simulink model "pid"  (R2022a)
settings: Solver=VariableStepAuto  StartTime=0  StopTime=15  RelTol=1e-3
libraries: slpidlib x3
settings Model: Creator=yfx13  LastModifiedBy=yfx13

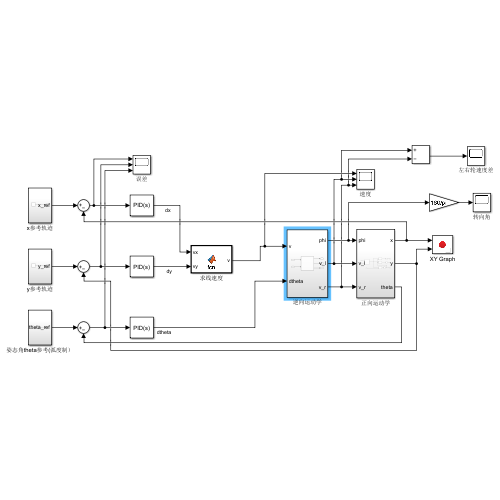
[thumbnail: Simulink's stored preview of the top-level diagram]
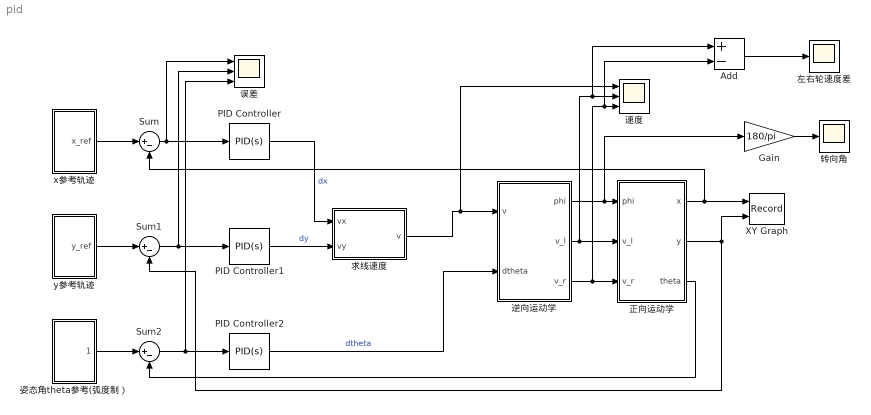
== system pid ==
  Add : Sum  Inputs=+-
  Gain : Gain  Gain=180/pi
  PID Controller : slpidlib/PID Controller  Controller=PID  Form=Parallel  TimeDomain=Continuous-time  UseExternalTs=off  SampleTime=-1  IntegratorMethod=Forward Euler  FilterMethod=Forward Euler  ControllerParametersSource=internal  P=11.7  I=0.72  UseKiTs=off  D=0.86  N=100  UseFilter=on  TunerSelectOption=Transfer Function Based (PID Tuner App)  InitialConditionSource=internal  InitialConditionForIntegrator=0  InitialConditionForFilter=0  DifferentiatorICPrevScaledInput=0  ExternalReset=none  TrackingMode=off  Kt=1  LimitOutput=off  SatLimitsSource=internal  UpperSaturationLimit=inf  LowerSaturationLimit=-inf  LinearizeAsGain=on  AntiWindupMode=none  Kb=1  POutMin=[]  POutMax=[]  IOutMin=[]  IOutMax=[]  DOutMin=[]  DOutMax=[]  NOutMin=[]  NOutMax=[]  SumOutMin=[]  SumOutMax=[]  SaturationOutMin=[]  SaturationOutMax=[]  PParamMin=[]  PParamMax=[]  IParamMin=[]  IParamMax=[]  DParamMin=[]  DParamMax=[]  NParamMin=[]  NParamMax=[]  KbParamMin=[]  KbParamMax=[]  KtParamMin=[]  KtParamMax=[]  KbOutMin=[]  KbOutMax=[]  KtOutMin=[]  KtOutMax=[]  IntegratorOutMin=[]  IntegratorOutMax=[]  FilterOutMin=[]  FilterOutMax=[]  SumI1OutMin=[]  SumI1OutMax=[]  SumI2OutMin=[]  SumI2OutMax=[]  SumI3OutMin=[]  SumI3OutMax=[]  SumI4OutMin=[]  SumI4OutMax=[]  SumDOutMin=[]  SumDOutMax=[]  DifferentiatorOutMin=[]  DifferentiatorOutMax=[]  FilterDiffOutCoefMin=[]  FilterDiffOutCoefMax=[]  ReciprocalOutMin=[]  ReciprocalOutMax=[]  SumDenOutMin=[]  SumDenOutMax=[]  SumNumOutMin=[]  SumNumOutMax=[]  DivideOutMin=[]  DivideOutMax=[]  UdiffTsProdOutMin=[]  UdiffTsProdOutMax=[]  NTsProdOutMin=[]  NTsProdOutMax=[]  UintegralTsProdOutMin=[]  UintegralTsProdOutMax=[]  UngainTsProdOutMin=[]  UngainTsProdOutMax=[]  IntegratorContinuousStateAttributes=''  IntegratorStateMustResolveToSignalObject=off  IntegratorRTWStateStorageClass=Auto  FilterContinuousStateAttributes=''  FilterStateMustResolveToSignalObject=off  FilterRTWStateStorageClass=Auto  ParallelPVariant=InternalParameters  IdealPVariant=Disabled  IVariant=InternalParameters  DVariant=InternalParameters  IntegratorVariant=Continuous  SatVariant=Disabled  AWVariant=Passthrough  PCopyVariant=Disabled  TRVariant=Disabled  FdbkBlocksVariant=Forward  IdealPFdbkVariant=Disabled  SatFdbkVariant=Disabled  DerivativeFilterVariant=ContFilter  NVariant=InternalParameters  NCopyVariant=Disabled  FilterICVariant=InternalICsFilter  IntegratorICVariant=InternalICs  ExternalResetVariant=Disabled  TRSumVariant=Passthrough  SumFdbkVariant=Disabled  SumVariant=Sum_PID  TsampFilterVariant=InternalTs  TsampNgainVariant=Passthrough  TsampIntegralVariant=Passthrough  ExternalSaturationOutDataTypeStr=Inherit: Same as second input  aMode=0
  PID Controller1 : slpidlib/PID Controller  Controller=PID  Form=Parallel  TimeDomain=Continuous-time  UseExternalTs=off  SampleTime=-1  IntegratorMethod=Forward Euler  FilterMethod=Forward Euler  ControllerParametersSource=internal  P=11.6  I=0.63  UseKiTs=off  D=0.78  N=100  UseFilter=on  TunerSelectOption=Transfer Function Based (PID Tuner App)  InitialConditionSource=internal  InitialConditionForIntegrator=0  InitialConditionForFilter=0  DifferentiatorICPrevScaledInput=0  ExternalReset=none  TrackingMode=off  Kt=1  LimitOutput=off  SatLimitsSource=internal  UpperSaturationLimit=inf  LowerSaturationLimit=-inf  LinearizeAsGain=on  AntiWindupMode=none  Kb=1  POutMin=[]  POutMax=[]  IOutMin=[]  IOutMax=[]  DOutMin=[]  DOutMax=[]  NOutMin=[]  NOutMax=[]  SumOutMin=[]  SumOutMax=[]  SaturationOutMin=[]  SaturationOutMax=[]  PParamMin=[]  PParamMax=[]  IParamMin=[]  IParamMax=[]  DParamMin=[]  DParamMax=[]  NParamMin=[]  NParamMax=[]  KbParamMin=[]  KbParamMax=[]  KtParamMin=[]  KtParamMax=[]  KbOutMin=[]  KbOutMax=[]  KtOutMin=[]  KtOutMax=[]  IntegratorOutMin=[]  IntegratorOutMax=[]  FilterOutMin=[]  FilterOutMax=[]  SumI1OutMin=[]  SumI1OutMax=[]  SumI2OutMin=[]  SumI2OutMax=[]  SumI3OutMin=[]  SumI3OutMax=[]  SumI4OutMin=[]  SumI4OutMax=[]  SumDOutMin=[]  SumDOutMax=[]  DifferentiatorOutMin=[]  DifferentiatorOutMax=[]  FilterDiffOutCoefMin=[]  FilterDiffOutCoefMax=[]  ReciprocalOutMin=[]  ReciprocalOutMax=[]  SumDenOutMin=[]  SumDenOutMax=[]  SumNumOutMin=[]  SumNumOutMax=[]  DivideOutMin=[]  DivideOutMax=[]  UdiffTsProdOutMin=[]  UdiffTsProdOutMax=[]  NTsProdOutMin=[]  NTsProdOutMax=[]  UintegralTsProdOutMin=[]  UintegralTsProdOutMax=[]  UngainTsProdOutMin=[]  UngainTsProdOutMax=[]  IntegratorContinuousStateAttributes=''  IntegratorStateMustResolveToSignalObject=off  IntegratorRTWStateStorageClass=Auto  FilterContinuousStateAttributes=''  FilterStateMustResolveToSignalObject=off  FilterRTWStateStorageClass=Auto  ParallelPVariant=InternalParameters  IdealPVariant=Disabled  IVariant=InternalParameters  DVariant=InternalParameters  IntegratorVariant=Continuous  SatVariant=Disabled  AWVariant=Passthrough  PCopyVariant=Disabled  TRVariant=Disabled  FdbkBlocksVariant=Forward  IdealPFdbkVariant=Disabled  SatFdbkVariant=Disabled  DerivativeFilterVariant=ContFilter  NVariant=InternalParameters  NCopyVariant=Disabled  FilterICVariant=InternalICsFilter  IntegratorICVariant=InternalICs  ExternalResetVariant=Disabled  TRSumVariant=Passthrough  SumFdbkVariant=Disabled  SumVariant=Sum_PID  TsampFilterVariant=InternalTs  TsampNgainVariant=Passthrough  TsampIntegralVariant=Passthrough  ExternalSaturationOutDataTypeStr=Inherit: Same as second input  aMode=0
  PID Controller2 : slpidlib/PID Controller  Controller=PID  Form=Parallel  TimeDomain=Continuous-time  UseExternalTs=off  SampleTime=-1  IntegratorMethod=Forward Euler  FilterMethod=Forward Euler  ControllerParametersSource=internal  P=10.3  I=2.86  UseKiTs=off  D=0.028  N=100  UseFilter=on  TunerSelectOption=Transfer Function Based (PID Tuner App)  InitialConditionSource=internal  InitialConditionForIntegrator=0.001  InitialConditionForFilter=0  DifferentiatorICPrevScaledInput=0  ExternalReset=none  TrackingMode=off  Kt=1  LimitOutput=off  SatLimitsSource=internal  UpperSaturationLimit=inf  LowerSaturationLimit=-inf  LinearizeAsGain=on  AntiWindupMode=none  Kb=1  POutMin=[]  POutMax=[]  IOutMin=[]  IOutMax=[]  DOutMin=[]  DOutMax=[]  NOutMin=[]  NOutMax=[]  SumOutMin=[]  SumOutMax=[]  SaturationOutMin=[]  SaturationOutMax=[]  PParamMin=[]  PParamMax=[]  IParamMin=[]  IParamMax=[]  DParamMin=[]  DParamMax=[]  NParamMin=[]  NParamMax=[]  KbParamMin=[]  KbParamMax=[]  KtParamMin=[]  KtParamMax=[]  KbOutMin=[]  KbOutMax=[]  KtOutMin=[]  KtOutMax=[]  IntegratorOutMin=[]  IntegratorOutMax=[]  FilterOutMin=[]  FilterOutMax=[]  SumI1OutMin=[]  SumI1OutMax=[]  SumI2OutMin=[]  SumI2OutMax=[]  SumI3OutMin=[]  SumI3OutMax=[]  SumI4OutMin=[]  SumI4OutMax=[]  SumDOutMin=[]  SumDOutMax=[]  DifferentiatorOutMin=[]  DifferentiatorOutMax=[]  FilterDiffOutCoefMin=[]  FilterDiffOutCoefMax=[]  ReciprocalOutMin=[]  ReciprocalOutMax=[]  SumDenOutMin=[]  SumDenOutMax=[]  SumNumOutMin=[]  SumNumOutMax=[]  DivideOutMin=[]  DivideOutMax=[]  UdiffTsProdOutMin=[]  UdiffTsProdOutMax=[]  NTsProdOutMin=[]  NTsProdOutMax=[]  UintegralTsProdOutMin=[]  UintegralTsProdOutMax=[]  UngainTsProdOutMin=[]  UngainTsProdOutMax=[]  IntegratorContinuousStateAttributes=''  IntegratorStateMustResolveToSignalObject=off  IntegratorRTWStateStorageClass=Auto  FilterContinuousStateAttributes=''  FilterStateMustResolveToSignalObject=off  FilterRTWStateStorageClass=Auto  ParallelPVariant=InternalParameters  IdealPVariant=Disabled  IVariant=InternalParameters  DVariant=InternalParameters  IntegratorVariant=Continuous  SatVariant=Disabled  AWVariant=Passthrough  PCopyVariant=Disabled  TRVariant=Disabled  FdbkBlocksVariant=Forward  IdealPFdbkVariant=Disabled  SatFdbkVariant=Disabled  DerivativeFilterVariant=ContFilter  NVariant=InternalParameters  NCopyVariant=Disabled  FilterICVariant=InternalICsFilter  IntegratorICVariant=InternalICs  ExternalResetVariant=Disabled  TRSumVariant=Passthrough  SumFdbkVariant=Disabled  SumVariant=Sum_PID  TsampFilterVariant=InternalTs  TsampNgainVariant=Passthrough  TsampIntegralVariant=Passthrough  ExternalSaturationOutDataTypeStr=Inherit: Same as second input  aMode=0
  Sum : Sum  Inputs=|+-
  Sum1 : Sum  Inputs=|+-
  Sum2 : Sum  Inputs=|+-
  XY Graph : Record  FileSettingsInternal="{\"entries\":[{\"content\":{\"excelSettings\":{\"content\":{},\"type\":\"Streamout.ExcelSettings\"}},\"type\":\"Streamout.FileSettingStorage\",\"uuid\":\"fc5dee4a-28b3-4ad2-9bcc-4b5cd185ba70\"}],\"packageUris\":[\"http://schema.mathworks.com/mf0/streamout_blocks/R2020a\"],\"version\":\"1.0\"}"  Layout=[1 1]  SignalsInternal="{\"entries\":[{\"content\":{\"signals\":[{\"content\":{\"blockPath\":[\"test/XY Graph\"],\"channel\":[],\"dimensions\":[1],\"domain\":\"test/XY Graph\",\"lineColor\":\"#a2142f\",\"plots\":[1],\"port\":1,\"sid\":[\"\"],\"signalID\":3670,\"signalName\":\"正向运动学:1\"},\"type\":\"RecordBlkView.Signal\",\"uuid\":\"a53176e7-da72-4e25-9eef-323f38d3bce5\"},{\"content\":{\"blockPath\":[\"test/XY Graph\"],\"channel\":[],\"dimensions\":[1],\"domain\":\"test/XY Graph\",\"lineColor\":\"#139fff\",\"plots\":[1],\"port\":2,\"sid\":[\"\"],\"signalID\":3674,\"signalName\":\"正向运动学:2\"},\"type\":\"RecordBlkView.Signal\",\"uuid\":\"ea951a5b-6c87-4f27-a4cb-4083dd1a02af\"}]},\"type\":\"RecordBlkView.InputSignals\",\"uuid\":\"8d8d5ef0-8d8d-4bbe-b956-2a655789d6ca\"}],\"packageUris\":[\"http://schema.mathworks.com/mf0/streamout_blocks/R2020a\"],\"version\":\"1.0\"}"  VisualizationBindings="{\"xyplotplugin\":{\"info\":[{\"series\":[{\"bindingParametersList\":[{\"parameter\":\"X-Axis\",\"signalID\":3670,\"signalName\":\"正向运动学:1\"},{\"parameter\":\"Y-Axis\",\"signalID\":3674,\"signalName\":\"正向运动学:2\"}],\"seriesID\":62762}],\"subplotID\":1}]}}"  CompatibilityTag=XY
  x参考轨迹 : Subsystem
  y参考轨迹 : Subsystem
  姿态角theta参考(弧度制） : Subsystem
  左右轮速度差 : Scope
  正向运动学 : Subsystem
  求线速度 : MATLAB Function  TreatAsAtomicUnit=on
  误差 : Scope  NumInputPorts=3
  转向角 : Scope
  逆向运动学 : Subsystem
  速度 : Scope  NumInputPorts=3
  wires:
  Sum/1 -> 误差/1, PID Controller/1
  x参考轨迹/1(x_ref) -> Sum/1
  PID Controller/1 -> 求线速度/1(vx)  "dx"
  Sum1/1 -> 误差/2, PID Controller1/1
  PID Controller1/1 -> 求线速度/2(vy)  "dy"
  y参考轨迹/1(y_ref) -> Sum1/1
  姿态角theta参考(弧度制）/1(theta_ref) -> Sum2/1
  Sum2/1 -> 误差/3, PID Controller2/1
  逆向运动学/1(phi) -> Gain/1, 正向运动学/1(phi)
  正向运动学/1(x) -> Sum/2, XY Graph/1
  正向运动学/2(y) -> Sum1/2, XY Graph/2
  正向运动学/3(theta) -> Sum2/2
  求线速度/1(v) -> 速度/1, 逆向运动学/1(v)
  PID Controller2/1 -> 逆向运动学/2(dtheta)  "dtheta"
  逆向运动学/2(v_l) -> Add/1, 速度/2, 正向运动学/2(v_l)
  Add/1 -> 左右轮速度差/1
  Gain/1 -> 转向角/1
  逆向运动学/3(v_r) -> Add/2, 速度/3, 正向运动学/3(v_r)

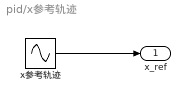
== system pid/x参考轨迹 ==
  x参考轨迹 : Sin  Amplitude=4  Frequency=pi/4  SampleTime=0
  x_ref : Outport
  wires:
  x参考轨迹/1 -> x_ref/1

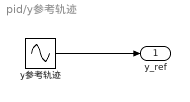
== system pid/y参考轨迹 ==
  y参考轨迹 : Sin  Amplitude=4  Bias=4  Frequency=pi/4  Phase=-pi/2  SampleTime=0
  y_ref : Outport
  wires:
  y参考轨迹/1 -> y_ref/1

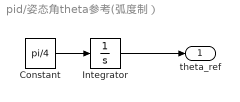
== system pid/姿态角theta参考(弧度制） ==
  Constant : Constant  Value=pi/4
  Integrator : Integrator
  theta_ref : Outport
  wires:
  Integrator/1 -> theta_ref/1
  Constant/1 -> Integrator/1

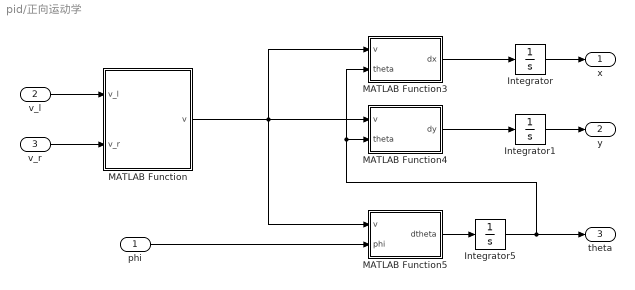
== system pid/正向运动学 ==
  phi : Inport
  v_l : Inport  Port=2
  v_r : Inport  Port=3
  Integrator : Integrator  InitialCondition=0.0001
  Integrator1 : Integrator
  Integrator5 : Integrator
  MATLAB Function : MATLAB Function  TreatAsAtomicUnit=on
  MATLAB Function3 : MATLAB Function  TreatAsAtomicUnit=on
  MATLAB Function4 : MATLAB Function  TreatAsAtomicUnit=on
  MATLAB Function5 : MATLAB Function  TreatAsAtomicUnit=on
  x : Outport
  y : Outport  Port=2
  theta : Outport  Port=3
  wires:
  MATLAB Function5/1(dtheta) -> Integrator5/1
  phi/1 -> MATLAB Function5/2(phi)
  MATLAB Function3/1(dx) -> Integrator/1
  Integrator/1 -> x/1
  Integrator1/1 -> y/1
  MATLAB Function4/1(dy) -> Integrator1/1
  Integrator5/1 -> MATLAB Function3/2(theta), MATLAB Function4/2(theta), theta/1
  MATLAB Function/1(v) -> MATLAB Function3/1(v), MATLAB Function5/1(v), MATLAB Function4/1(v)
  v_l/1 -> MATLAB Function/1(v_l)
  v_r/1 -> MATLAB Function/2(v_r)

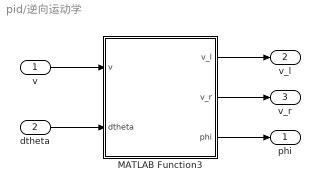
== system pid/逆向运动学 ==
  v : Inport
  dtheta : Inport  Port=2
  MATLAB Function3 : MATLAB Function  TreatAsAtomicUnit=on
  phi : Outport
  v_l : Outport  Port=2
  v_r : Outport  Port=3
  wires:
  dtheta/1 -> MATLAB Function3/2(dtheta)
  v/1 -> MATLAB Function3/1(v)
  MATLAB Function3/1(v_l) -> v_l/1
  MATLAB Function3/2(v_r) -> v_r/1
  MATLAB Function3/3(phi) -> phi/1

== matlab function pid/求线速度 ==
  data: vx input; v output; vy input
function v = fcn(vx,vy)

v = sqrt(vx^2+vy^2);

== matlab function pid/正向运动学/MATLAB Function3 ==
  data: v input; dx output; theta input
function dx = fcn(v,theta)
dx=v*cos(theta);

== matlab function pid/正向运动学/MATLAB Function4 ==
  data: v input; dy output; theta input
function dy = fcn(v,theta)
dy=v*sin(theta);

== matlab function pid/正向运动学/MATLAB Function5 ==
  data: v input; dtheta output; phi input
function dtheta = fcn(v,phi)
L=0.28;
dtheta=v*tan(phi)/L;

== matlab function pid/正向运动学/MATLAB Function ==
  data: v_l input; v output; v_r input
function v = fcn(v_l,v_r)
v=(v_l+v_r)/2;

== matlab function pid/逆向运动学/MATLAB Function3 ==
  data: v input; dtheta input; v_l output; v_r output; phi output
function [v_l,v_r,phi] = fcn(v,dtheta)
W=0.18;%宽度
L=0.28;
R=v/dtheta;   %L/phi;

v_l = (v/R)*(R-W/2);
v_r = (v/R)*(R+W/2);

phi_l=atan(L/(R-W/2));
phi_r=atan(L/(R+W/2));
phi=(phi_l+phi_r)/2;
if phi>pi/2
    phi=pi/2;
end
